simulink model "gm_homework1"  (R2020b)
settings: Solver=FixedStepDiscrete  StartTime=0.0  StopTime=simulation_stop_time  RelTol=1e-3
undefined symbols (not defined in the file or in its folder): sample_time
libraries: hdlsllib x4, simulink x3
settings Model: Creator=yixingli  LastModifiedBy=harsh
settings DataIOCC: LimitDataPoints=on  SaveOutput=off  SignalLogging=off  SaveTime=off
settings OptimizationCC: BlockReduction=off  ConditionallyExecuteInputs=off  DefaultParameterBehavior=Inlined  ExpressionDepthLimit=2147483647  LifeSpan=inf
settings DebuggingCC: AlgebraicLoopMsg=error  UnderspecifiedInitializationDetection=Classic  MergeDetectMultiDrivingBlocksExec=none  InheritedTsInSrcMsg=none  SingleTaskRateTransMsg=error  ParameterPrecisionLossMsg=none  AllowSymbolicDim=off  StateNameClashWarn=warning  StrictBusMsg=ErrorOnBusTreatedAsVector  SFUnexpectedBacktrackingDiag=warning  SFNoUnconditionalDefaultTransitionDiag=warning  SFExecutionAtInitializationDiag=none  ArithmeticOperatorsInVariantConditions=warning
settings HardwareCC: ProdBitPerPointer=32  ProdBitPerSizeT=32  ProdBitPerPtrDiffT=32  ProdLargestAtomicFloat=None  ProdIntDivRoundTo=Undefined  ProdEndianess=Unspecified  ProdWordSize=32  ProdHWDeviceType=ASIC/FPGA->ASIC/FPGA  ProdEqTarget=off
settings SFSimCC: SimUseLocalCustomCode=off  CustomCodeUndefinedFunction=UseInterfaceOnly
settings RTWCC: RTWUseLocalCustomCode=off
settings CodeAppCC: StateflowObjectComments=on
settings GRTTargetCC: TargetLangStandard=C89/C90 (ANSI)
settings ConfigComp: CovScope=ReferencedModels  CovMetricSettings=dw  CovSaveCumulativeToWorkspaceVar=on  CovSaveSingleToWorkspaceVar=on  CovExternalEMLEnable=off  CovSFcnEnable=off

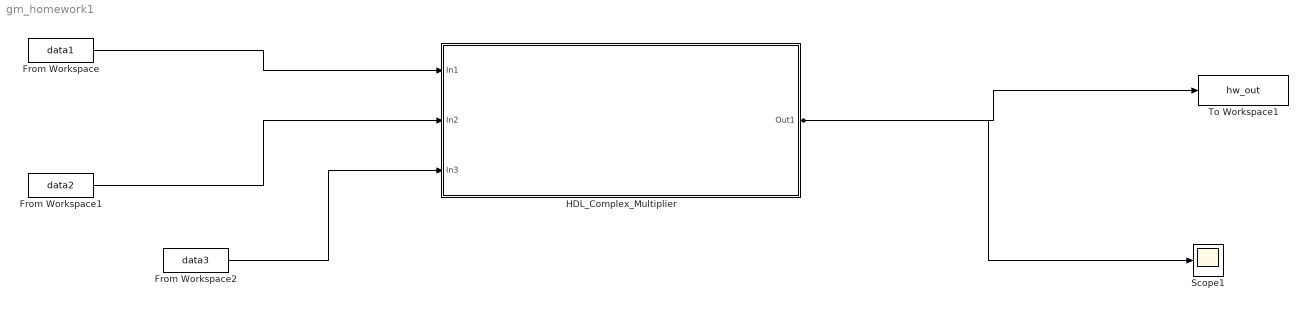
== system gm_homework1 ==
  From Workspace : FromWorkspace  VariableName=data1  SampleTime=sample_time  Interpolate=off  OutputAfterFinalValue=Setting to zero
  From Workspace1 : FromWorkspace  VariableName=data2  SampleTime=sample_time  Interpolate=off  OutputAfterFinalValue=Setting to zero
  From Workspace2 : FromWorkspace  VariableName=data3  SampleTime=sample_time  Interpolate=off  OutputAfterFinalValue=Setting to zero
  HDL_Complex_Multiplier : Subsystem
  Scope1 : Scope
  To Workspace1 : ToWorkspace  VariableName=hw_out  SaveFormat=Structure With Time  SampleTime=-1
  wires:
  From Workspace2/1 -> HDL_Complex_Multiplier/3(In3)
  HDL_Complex_Multiplier/1(Out1) -> Scope1/1, To Workspace1/1
  From Workspace1/1 -> HDL_Complex_Multiplier/2(In2)
  From Workspace/1 -> HDL_Complex_Multiplier/1(In1)

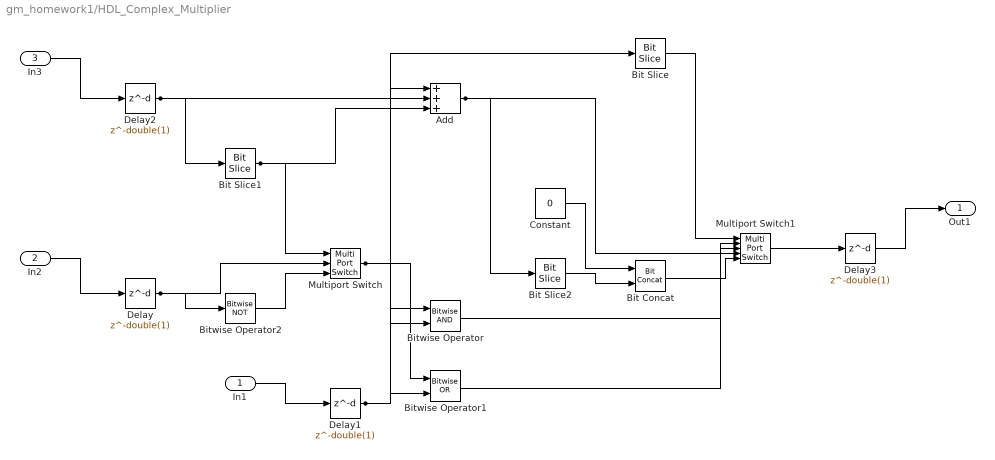
== system gm_homework1/HDL_Complex_Multiplier ==
  In1 : Inport  OutDataTypeStr=fixdt(1, 64, 0)  PortDimensions=1  SampleTime=5e-08
  In2 : Inport  Port=2  OutDataTypeStr=fixdt(1, 64, 0)  PortDimensions=1  SampleTime=5e-08
  In3 : Inport  Port=3  OutDataTypeStr=fixdt(0, 3, 0)  PortDimensions=1  SampleTime=5e-08
  Add : Sum  Inputs=+++  AccumDataTypeStr=fixdt(1, 65, 0)  OutDataTypeStr=fixdt(1, 64, 0)  SampleTime=5e-08
  Bit Concat : hdlsllib/Logic and Bit Operations/Bit Concat  numInputs=2
  Bit Slice : hdlsllib/Logic and Bit Operations/Bit Slice  lidx=double(1)  ridx=double(0)
      settings: SourceProductBaseCode=SL
  Bit Slice1 : hdlsllib/Logic and Bit Operations/Bit Slice  lidx=double(2)  ridx=double(2)
      settings: SourceProductBaseCode=SL
  Bit Slice2 : hdlsllib/Logic and Bit Operations/Bit Slice  lidx=double(62)  ridx=double(62)
      settings: SourceProductBaseCode=SL
  Bitwise Operator : simulink/Logic and Bit Operations/Bitwise Operator  logicop=AND  UseBitMask=off  NumInputPorts=2  BitMask=double(0)  BitMaskRealWorld=Real World Value
  Bitwise Operator1 : simulink/Logic and Bit Operations/Bitwise Operator  logicop=OR  UseBitMask=off  NumInputPorts=2  BitMask=double(0)  BitMaskRealWorld=Real World Value
  Bitwise Operator2 : simulink/Logic and Bit Operations/Bitwise Operator  logicop=NOT  UseBitMask=off  BitMask=double(0)  BitMaskRealWorld=Real World Value
  Constant : Constant  Value=0  OutDataTypeStr=fixdt(0, 64, 0)
  Delay{,1..3} (4 alike) : Delay  DelayLength=double(1)  InitialCondition=0  SampleTime=5e-08
  Multiport Switch : MultiPortSwitch  DataPortOrder=Zero-based contiguous  Inputs=2  DiagnosticForDefault=None  zeroidx=on  OutDataTypeStr=fixdt(1, 64, 0)  SampleTime=5e-08
  Multiport Switch1 : MultiPortSwitch  DataPortOrder=Zero-based contiguous  Inputs=4  DiagnosticForDefault=None  zeroidx=on  OutDataTypeStr=fixdt(1, 64, 0)  SampleTime=5e-08
  Out1 : Outport
  wires:
  In1/1 -> Delay1/1
  In2/1 -> Delay/1
  In3/1 -> Delay2/1
  Add/1 -> Multiport Switch1/4, Bit Slice2/1
  Bit Concat/1 -> Multiport Switch1/5
  Bit Slice/1 -> Multiport Switch1/1
  Bit Slice1/1 -> Multiport Switch/1, Add/3
  Bit Slice2/1 -> Bit Concat/2
  Bitwise Operator/1 -> Multiport Switch1/2
  Bitwise Operator1/1 -> Multiport Switch1/3
  Bitwise Operator2/1 -> Multiport Switch/3
  Constant/1 -> Bit Concat/1
  Delay/1 -> Multiport Switch/2, Bitwise Operator2/1
  Delay1/1 -> Bitwise Operator1/2, Bitwise Operator/2, Add/2
  Delay2/1 -> Bit Slice1/1, Bit Slice/1
  Delay3/1 -> Out1/1
  Multiport Switch/1 -> Bitwise Operator1/1, Bitwise Operator/1, Add/1
  Multiport Switch1/1 -> Delay3/1
